simulink subsystem "rss_PhCurrSensFaltDia"  (R2023a)
settings: Solver=VariableStepAuto  StartTime=0.0  StopTime=10.0  RelTol=1e-3
undefined symbols (not defined in the file): ENM_TYPE_FALT, Gu16_ctPhCurrSensFaltConfCnt_C, Gu16_ctPhCurrSensFaltRcvyCnt_C, Gu16_uADPhUCurrFaltHiLim_C, Gu16_uADPhUCurrFaltLoLim_C, Gu16_uADPhVCurrFaltHiLim_C, Gu16_uADPhVCurrFaltLoLim_C
libraries: lib_debounce x1, lib_fault_definiteness x1
settings Model: Creator=xiaoqiang.yuan  LastModifiedBy=xiaoqiang.yuan

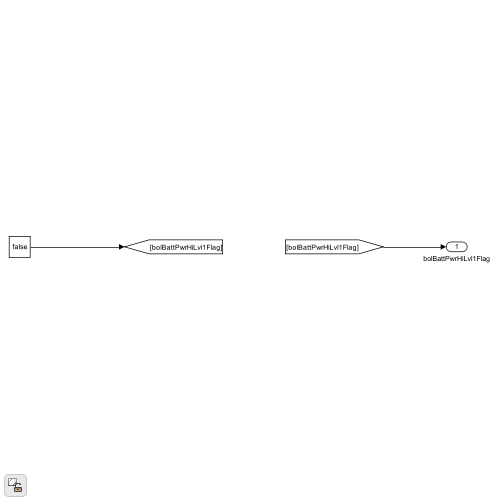
[thumbnail: Simulink's stored preview of the top-level diagram]
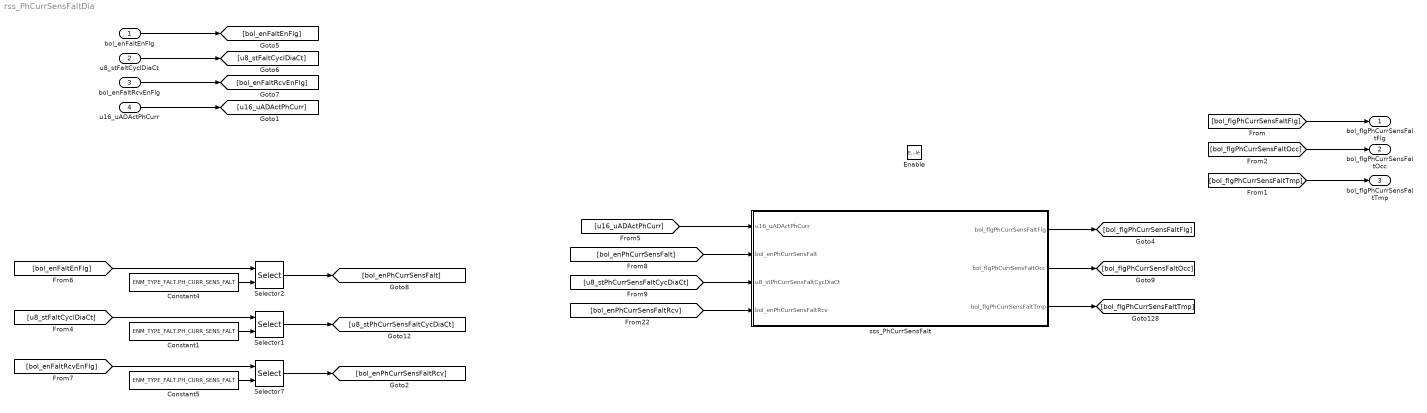
== system rss_PhCurrSensFaltDia ==
  bol_enFaltEnFlg : Inport  OutDataTypeStr=boolean
  u8_stFaltCyclDiaCt : Inport  Port=2  OutDataTypeStr=uint8
  bol_enFaltRcvEnFlg : Inport  Port=3  OutDataTypeStr=boolean
  u16_uADActPhCurr : Inport  Port=4  OutDataTypeStr=uint16
  Enable : EnablePort
  Constant1 : Constant  Value=ENM_TYPE_FALT.PH_CURR_SENS_FALT
  Constant4 : Constant  Value=ENM_TYPE_FALT.PH_CURR_SENS_FALT
  Constant5 : Constant  Value=ENM_TYPE_FALT.PH_CURR_SENS_FALT
  Selector1 : Selector  IndexMode=Zero-based  InputPortWidth=Cdbl_numFaltDiaNum  IndexOptions=Index vector (port)  Indices=[1 3]  OutputSizes=1
  Selector2 : Selector  IndexMode=Zero-based  InputPortWidth=Cdbl_numFaltDiaNum  IndexOptions=Index vector (port)  Indices=[1 3]  OutputSizes=1
  Selector7 : Selector  IndexMode=Zero-based  InputPortWidth=Cdbl_numFaltDiaNum  IndexOptions=Index vector (port)  Indices=[1 3]  OutputSizes=1
  sss_PhCurrSensFalt : Subsystem
  bol_flgPhCurrSensFaltFlg : Outport  OutDataTypeStr=boolean
  bol_flgPhCurrSensFaltOcc : Outport  Port=2  OutDataTypeStr=boolean
  bol_flgPhCurrSensFaltTmp : Outport  Port=3  OutDataTypeStr=boolean
  wires:
  [bol_flgPhCurrSensFaltFlg] -> bol_flgPhCurrSensFaltFlg/1
  Selector1/1 -> [u8_stPhCurrSensFaltCycDiaCt]
  [bol_enPhCurrSensFalt] -> sss_PhCurrSensFalt/2(bol_enPhCurrSensFalt)
  sss_PhCurrSensFalt/1(bol_flgPhCurrSensFaltFlg) -> [bol_flgPhCurrSensFaltFlg]
  bol_enFaltRcvEnFlg/1 -> [bol_enFaltRcvEnFlg]
  u16_uADActPhCurr/1 -> [u16_uADActPhCurr]
  [bol_flgPhCurrSensFaltOcc] -> bol_flgPhCurrSensFaltOcc/1
  bol_enFaltEnFlg/1 -> [bol_enFaltEnFlg]
  [bol_enFaltEnFlg] -> Selector2/1
  [bol_enFaltRcvEnFlg] -> Selector7/1
  [u8_stPhCurrSensFaltCycDiaCt] -> sss_PhCurrSensFalt/3(u8_stPhCurrSensFaltCycDiaCt)
  Selector2/1 -> [bol_enPhCurrSensFalt]
  Selector7/1 -> [bol_enPhCurrSensFaltRcv]
  Constant4/1 -> Selector2/2
  sss_PhCurrSensFalt/2(bol_flgPhCurrSensFaltOcc) -> [bol_flgPhCurrSensFaltOcc]
  [u8_stFaltCyclDiaCt] -> Selector1/1
  Constant1/1 -> Selector1/2
  [bol_enPhCurrSensFaltRcv] -> sss_PhCurrSensFalt/4(bol_enPhCurrSensFaltRcv)
  [u16_uADActPhCurr] -> sss_PhCurrSensFalt/1(u16_uADActPhCurr)
  Constant5/1 -> Selector7/2
  u8_stFaltCyclDiaCt/1 -> [u8_stFaltCyclDiaCt]
  [bol_flgPhCurrSensFaltTmp] -> bol_flgPhCurrSensFaltTmp/1
  sss_PhCurrSensFalt/3(bol_flgPhCurrSensFaltTmp) -> [bol_flgPhCurrSensFaltTmp]

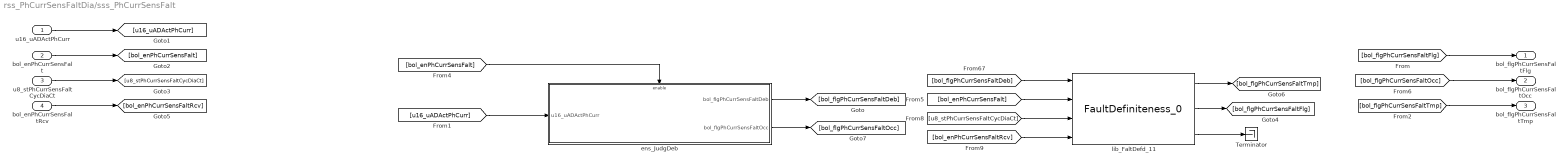
== system rss_PhCurrSensFaltDia/sss_PhCurrSensFalt ==
  u16_uADActPhCurr : Inport
  bol_enPhCurrSensFalt : Inport  Port=2
  u8_stPhCurrSensFaltCycDiaCt : Inport  Port=3
  bol_enPhCurrSensFaltRcv : Inport  Port=4
  Terminator : Terminator
  ens_JudgDeb : Subsystem
  lib_FaltDefd_11 : lib_fault_definiteness/FaultDefiniteness_0  lb_FaltWaitRecvCnt=Gu16_ctPhCurrSensFaltConfCnt_C
  bol_flgPhCurrSensFaltFlg : Outport
  bol_flgPhCurrSensFaltOcc : Outport  Port=2
  bol_flgPhCurrSensFaltTmp : Outport  Port=3
  wires:
  [bol_flgPhCurrSensFaltTmp] -> bol_flgPhCurrSensFaltTmp/1
  [bol_flgPhCurrSensFaltOcc] -> bol_flgPhCurrSensFaltOcc/1
  ens_JudgDeb/2(bol_flgPhCurrSensFaltOcc) -> [bol_flgPhCurrSensFaltOcc]
  lib_FaltDefd_11/1 -> [bol_flgPhCurrSensFaltTmp]
  lib_FaltDefd_11/2 -> [bol_flgPhCurrSensFaltFlg]
  lib_FaltDefd_11/3 -> Terminator/1
  [bol_enPhCurrSensFalt] -> ens_JudgDeb/Enable
  [u16_uADActPhCurr] -> ens_JudgDeb/1(u16_uADActPhCurr)
  ens_JudgDeb/1(bol_flgPhCurrSensFaltDeb) -> [bol_flgPhCurrSensFaltDeb]
  bol_enPhCurrSensFaltRcv/1 -> [bol_enPhCurrSensFaltRcv]
  u8_stPhCurrSensFaltCycDiaCt/1 -> [u8_stPhCurrSensFaltCycDiaCt]
  bol_enPhCurrSensFalt/1 -> [bol_enPhCurrSensFalt]
  [bol_flgPhCurrSensFaltFlg] -> bol_flgPhCurrSensFaltFlg/1
  u16_uADActPhCurr/1 -> [u16_uADActPhCurr]
  [bol_enPhCurrSensFaltRcv] -> lib_FaltDefd_11/4
  [u8_stPhCurrSensFaltCycDiaCt] -> lib_FaltDefd_11/3
  [bol_enPhCurrSensFalt] -> lib_FaltDefd_11/2
  [bol_flgPhCurrSensFaltDeb] -> lib_FaltDefd_11/1

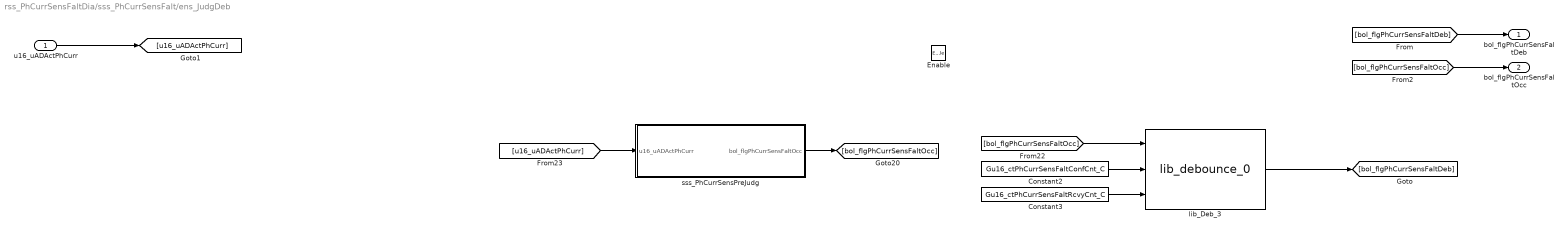
== system rss_PhCurrSensFaltDia/sss_PhCurrSensFalt/ens_JudgDeb ==
  u16_uADActPhCurr : Inport
  Enable : EnablePort
  Constant2 : Constant  Value=Gu16_ctPhCurrSensFaltConfCnt_C
  Constant3 : Constant  Value=Gu16_ctPhCurrSensFaltRcvyCnt_C
  lib_Deb_3 : lib_debounce/lib_debounce_0
  sss_PhCurrSensPreJudg : Subsystem
  bol_flgPhCurrSensFaltDeb : Outport
  bol_flgPhCurrSensFaltOcc : Outport  Port=2
  wires:
  [bol_flgPhCurrSensFaltOcc] -> bol_flgPhCurrSensFaltOcc/1
  [u16_uADActPhCurr] -> sss_PhCurrSensPreJudg/1(u16_uADActPhCurr)
  u16_uADActPhCurr/1 -> [u16_uADActPhCurr]
  [bol_flgPhCurrSensFaltDeb] -> bol_flgPhCurrSensFaltDeb/1
  sss_PhCurrSensPreJudg/1(bol_flgPhCurrSensFaltOcc) -> [bol_flgPhCurrSensFaltOcc]
  Constant3/1 -> lib_Deb_3/3
  [bol_flgPhCurrSensFaltOcc] -> lib_Deb_3/1
  lib_Deb_3/1 -> [bol_flgPhCurrSensFaltDeb]
  Constant2/1 -> lib_Deb_3/2

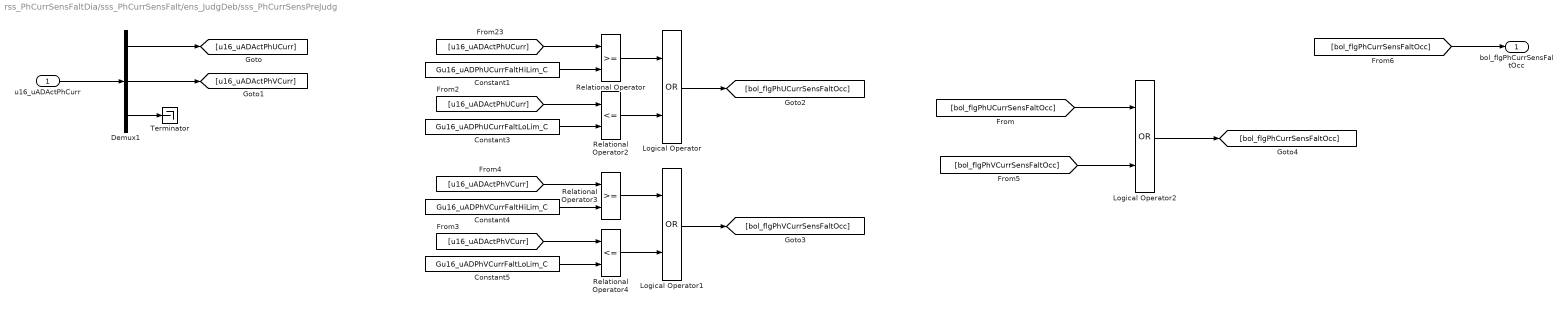
== system rss_PhCurrSensFaltDia/sss_PhCurrSensFalt/ens_JudgDeb/sss_PhCurrSensPreJudg ==
  u16_uADActPhCurr : Inport
  Constant1 : Constant  Value=Gu16_uADPhUCurrFaltHiLim_C
  Constant3 : Constant  Value=Gu16_uADPhUCurrFaltLoLim_C
  Constant4 : Constant  Value=Gu16_uADPhVCurrFaltHiLim_C
  Constant5 : Constant  Value=Gu16_uADPhVCurrFaltLoLim_C
  Demux1 : Demux  Outputs=3
  Logical Operator : Logic  Operator=OR  AllPortsSameDT=off  OutDataTypeStr=boolean
  Logical Operator1 : Logic  Operator=OR  AllPortsSameDT=off  OutDataTypeStr=boolean
  Logical Operator2 : Logic  Operator=OR  AllPortsSameDT=off  OutDataTypeStr=boolean
  Relational Operator : RelationalOperator  OutDataTypeStr=boolean  RndMeth=Simplest  InputSameDT=off
  Relational Operator2 : RelationalOperator  Operator=<=  OutDataTypeStr=boolean  RndMeth=Simplest  InputSameDT=off
  Relational Operator3 : RelationalOperator  OutDataTypeStr=boolean  RndMeth=Simplest  InputSameDT=off
  Relational Operator4 : RelationalOperator  Operator=<=  OutDataTypeStr=boolean  RndMeth=Simplest  InputSameDT=off
  Terminator : Terminator
  bol_flgPhCurrSensFaltOcc : Outport
  wires:
  [bol_flgPhCurrSensFaltOcc] -> bol_flgPhCurrSensFaltOcc/1
  Logical Operator2/1 -> [bol_flgPhCurrSensFaltOcc]
  [bol_flgPhVCurrSensFaltOcc] -> Logical Operator2/2
  [bol_flgPhUCurrSensFaltOcc] -> Logical Operator2/1
  Constant4/1 -> Relational Operator3/2
  Logical Operator1/1 -> [bol_flgPhVCurrSensFaltOcc]
  Relational Operator4/1 -> Logical Operator1/2
  [u16_uADActPhVCurr] -> Relational Operator3/1
  Constant5/1 -> Relational Operator4/2
  [u16_uADActPhVCurr] -> Relational Operator4/1
  Relational Operator3/1 -> Logical Operator1/1
  Logical Operator/1 -> [bol_flgPhUCurrSensFaltOcc]
  Relational Operator2/1 -> Logical Operator/2
  Relational Operator/1 -> Logical Operator/1
  [u16_uADActPhUCurr] -> Relational Operator2/1
  Constant3/1 -> Relational Operator2/2
  Constant1/1 -> Relational Operator/2
  [u16_uADActPhUCurr] -> Relational Operator/1
  Demux1/1 -> [u16_uADActPhUCurr]
  u16_uADActPhCurr/1 -> Demux1/1
  Demux1/3 -> Terminator/1
  Demux1/2 -> [u16_uADActPhVCurr]
